simulink model "hw10"
settings: Solver=ode45  StartTime=0.0  StopTime=10.0  RelTol=1e-3
settings Model: Creator=bazkoale  LastModifiedBy=alex
settings DataIOCC: LimitDataPoints=on  SaveFormat=Array  ReturnWorkspaceOutputs=off
settings OptimizationCC: LifeSpan=inf  SimCompilerOptimization=Off
settings DebuggingCC: UnderspecifiedInitializationDetection=Classic  MergeDetectMultiDrivingBlocksExec=none  SolverPrmCheckMsg=warning  MultiTaskDSMMsg=warning  MultiTaskCondExecSysMsg=none  FcnCallInpInsideContextMsg=Enable All  FrameProcessingCompatibilityMsg=warning  StateNameClashWarn=warning  StrictBusMsg=None  SFUnexpectedBacktrackingDiag=warning  SFNoUnconditionalDefaultTransitionDiag=warning
settings HardwareCC: ProdBitPerPointer=32  ProdLargestAtomicFloat=None  ProdIntDivRoundTo=Undefined  ProdEndianess=Unspecified  ProdWordSize=32  ProdHWDeviceType=32-bit Generic
settings ModelReferenceCC: PropagateSignalLabelsOutOfModel=off
settings SFSimCC: SimUseLocalCustomCode=off
settings RTWCC: RTWUseLocalCustomCode=off  IncludeERTFirstTime=on  RTWCompilerOptimization=Off
settings GRTTargetCC: CodeReplacementLibrary=ANSI_C  GeneratePreprocessorConditionals=Disable all  CPPClassGenCompliant=off

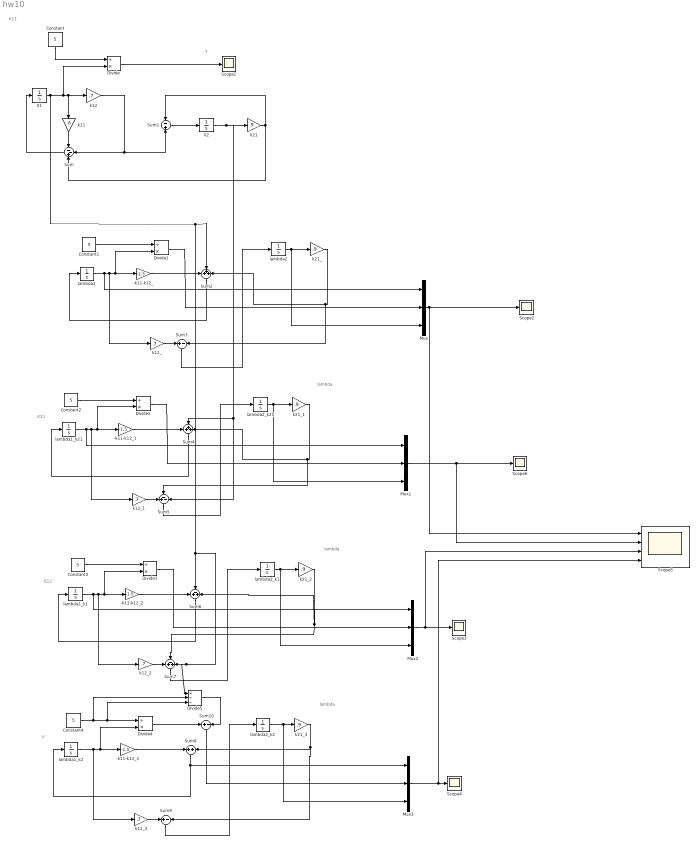
== system hw10 ==
  note: K21
  note: Y
  note: K11
  note: lambda
  note: K12
  note: lambda
  note: V
  note: lambda
  -k11-k12_{,1..3} (4 alike) : Gain  Gain=-1.5
  Constant{,1..4} (5 alike) : Constant  Value=5
  Divide{,1..4} (5 alike) : Product  Inputs=/*
  Divide5 : Product  Inputs=*//
  Mux{,1..3} (4 alike) : Mux  Inputs=3
  Scope{1..4,6} (5 alike) : Scope
      Scope2 settings: SaveName=ScopeData2
      Scope3 settings: SaveName=ScopeData3
      Scope4 settings: SaveName=ScopeData4
      Scope6 settings: SaveName=ScopeData5
  Scope5 : Scope  NumInputPorts=4
      settings: YMin=-5~-5~-5~-5  YMax=5~5~5~5
  Sum : Sum  Inputs=--+
  Sum1 : Sum  Inputs=-+
  Sum10 : Sum  Inputs=+|-
  Sum2 : Sum  Inputs=+++
  Sum3 : Sum  Inputs=+-
  Sum4 : Sum  Inputs=+++
  Sum5 : Sum  Inputs=+--
  Sum6 : Sum  Inputs=+-+
  Sum7 : Sum  Inputs=+-+
  Sum8 : Sum  Inputs=+|+
  Sum9 : Sum  Inputs=+|-
  X1 : Integrator  InitialCondition=200
  X2 : Integrator
  k11 : Gain  Gain=.8
  k12 : Gain  Gain=.7
  k12_{,1..3} (4 alike) : Gain  Gain=.7
  k21 : Gain  Gain=.9
  k21_{,1..3} (4 alike) : Gain  Gain=.9
  lambda1 : Integrator
  lambda1_k1 : Integrator
  lambda1_k2 : Integrator
  lambda1_k21 : Integrator
  lambda2 : Integrator
  lambda2_k1 : Integrator
  lambda2_k2 : Integrator
  lambda2_k21 : Integrator
  wires:
  X1/1 -> Divide/2, k11/1, k12/1, Sum2/2, Sum6/2, Sum7/3, Divide5/1
  k12/1 -> Sum1/2, Sum/2
  Sum/1 -> X1/1
  X2/1 -> k21/1, Sum4/2, Sum5/3
  Sum1/1 -> X2/1
  k21/1 -> Sum1/1, Sum/3
  k11/1 -> Sum/1
  Constant/1 -> Divide/1
  lambda1/1 -> Mux/1, Divide1/2, -k11-k12_/1, k12_/1
  -k11-k12_/1 -> Sum2/1
  lambda2/1 -> Mux/3, k21_/1
  k21_/1 -> Sum3/2, Sum2/3
  Constant1/1 -> Divide1/1
  Divide1/1 -> Mux/2
  Divide/1 -> Scope1/1
  Sum2/1 -> lambda1/1
  k12_/1 -> Sum3/1
  Sum3/1 -> lambda2/1
  lambda1_k21/1 -> Mux1/1, -k11-k12_1/1, Divide2/2, k12_1/1
  -k11-k12_1/1 -> Sum4/1
  lambda2_k21/1 -> k21_1/1, Mux1/3
  k21_1/1 -> Sum4/3, Sum5/2
  Constant2/1 -> Divide2/1
  Divide2/1 -> Mux1/2
  Sum4/1 -> lambda1_k21/1
  k12_1/1 -> Sum5/1
  Sum5/1 -> lambda2_k21/1
  lambda1_k1/1 -> k12_2/1, Divide3/2, -k11-k12_2/1, Mux2/1
  -k11-k12_2/1 -> Sum6/1
  lambda2_k1/1 -> Mux2/3, k21_2/1
  k21_2/1 -> Sum6/3, Sum7/2
  Mux2/1 -> Scope3/1, Scope5/3
  Constant3/1 -> Divide3/1
  Divide3/1 -> Mux2/2
  Sum6/1 -> lambda1_k1/1
  k12_2/1 -> Sum7/1
  Sum7/1 -> lambda2_k1/1
  lambda1_k2/1 -> -k11-k12_3/1, Divide4/2, k12_3/1
  -k11-k12_3/1 -> Sum8/1
  lambda2_k2/1 -> k21_3/1, Mux3/3
  k21_3/1 -> Sum9/2, Sum8/2
  Mux3/1 -> Scope4/1, Scope5/4
  Constant4/1 -> Divide5/2, Divide4/1, Divide5/3
  Sum8/1 -> lambda1_k2/1, Mux3/1
  k12_3/1 -> Sum9/1
  Sum9/1 -> lambda2_k2/1
  Divide4/1 -> Sum10/1
  Divide5/1 -> Sum10/2
  Sum10/1 -> Mux3/2
  Mux1/1 -> Scope6/1, Scope5/2
  Mux/1 -> Scope2/1, Scope5/1
